simulink model "LIF_Neuron"  (R2025a)
settings: Solver=ode45  StartTime=0.0  StopTime=0.5  FixedStep=1e-3  MaxStep=0.001  RelTol=1e-3
undefined symbols (not defined in the file): tau
libraries: eeGeneralControl x1
settings Model: Creator=pradipkumarde  LastModifiedBy=pradipkumarde

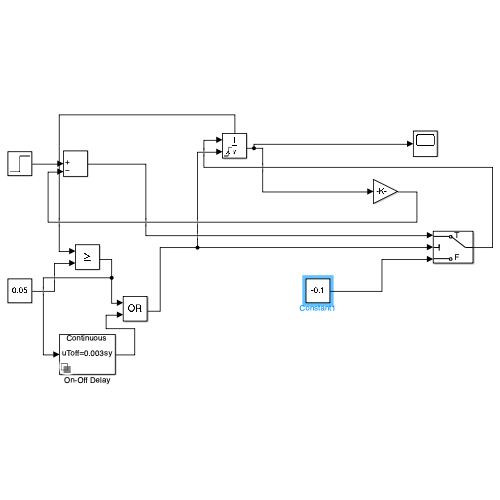
[thumbnail: Simulink's stored preview of the top-level diagram]
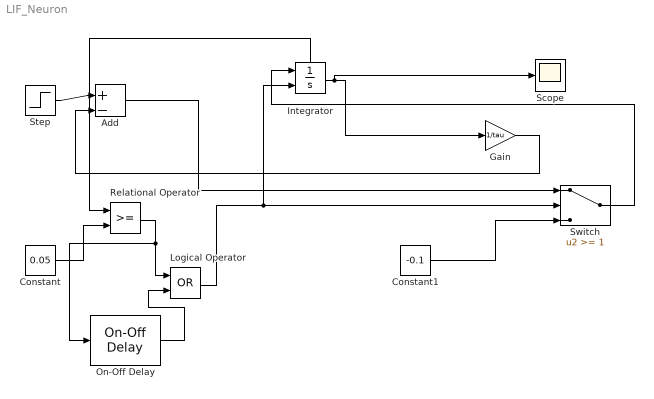
== system LIF_Neuron ==
  Add : Sum  Inputs=|+-
  Constant : Constant  Value=0.05
  Constant1 : Constant  Value=-0.1
  Gain : Gain  Gain=1/tau
  Integrator : Integrator  ExternalReset=rising  ShowStatePort=on
  Logical Operator : Logic  Operator=OR  AllPortsSameDT=off  OutDataTypeStr=boolean
  On-Off Delay : eeGeneralControl/On-Off Delay  LabelModeActiveChoice=Continuous  Td_on=0  Td_off=0.003  IC=0  Ts=0
      settings: LibrarySourceBlock=ee_sl_lib/General Control/On-Off Delay
  Relational Operator : RelationalOperator  OutDataTypeStr=boolean  RndMeth=Simplest  InputSameDT=off
  Scope : Scope
      settings: ActiveDisplayYMinimum=-1  ActiveDisplayYMaximum=1
  Step : Step  Time=0  After=5  SampleTime=0
  Switch : Switch  Threshold=1  SaturateOnIntegerOverflow=off  InputSameDT=off
  wires:
  Add/1 -> Switch/1
  Integrator/1 -> Gain/1, Scope/1
  Gain/1 -> Add/2
  Step/1 -> Add/1
  Relational Operator/1 -> On-Off Delay/1, Logical Operator/1
  Constant/1 -> Relational Operator/2
  Constant1/1 -> Switch/3
  Switch/1 -> Integrator/1
  On-Off Delay/1 -> Logical Operator/2
  Logical Operator/1 -> Integrator/2, Switch/2
  Integrator/State -> Relational Operator/1
